simulink model "brake_press_ex"  (R2023b)
settings: Solver=FixedStepAuto  StartTime=0.0  StopTime=10.0  FixedStep=0.01  RelTol=1e-3
settings Model: Creator=FM22  LastModifiedBy=FM22

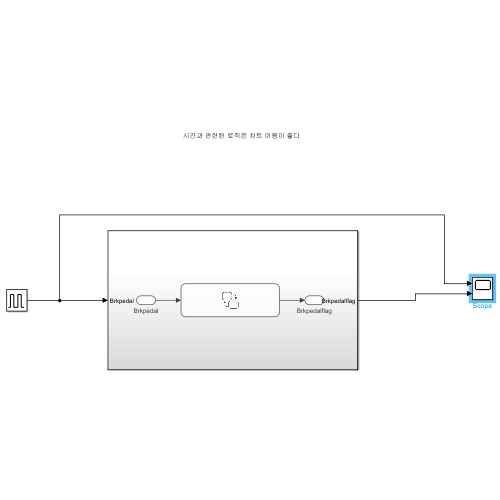
[thumbnail: Simulink's stored preview of the top-level diagram]
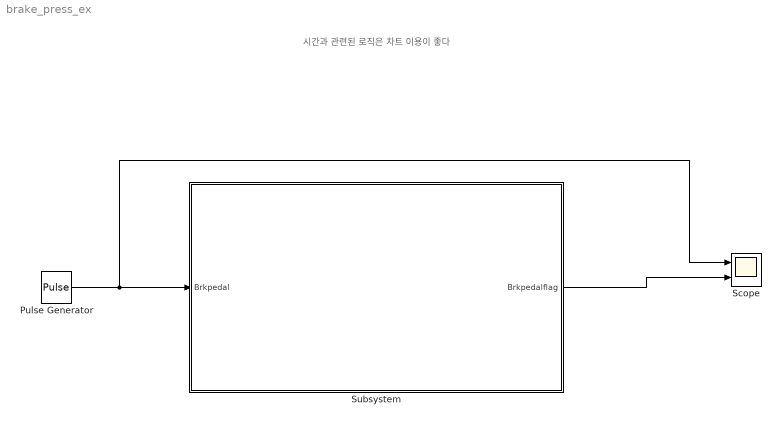
== system brake_press_ex ==
  note: 시간과 관련된 로직은 차트 이용이 좋다
  Pulse Generator : DiscretePulseGenerator  PulseType=Time based  Period=5  PulseWidth=50
  Scope : Scope  NumInputPorts=2
  Subsystem : Subsystem
  wires:
  Pulse Generator/1 -> Scope/1, Subsystem/1(Brkpedal)
  Subsystem/1(Brkpedalflag) -> Scope/2

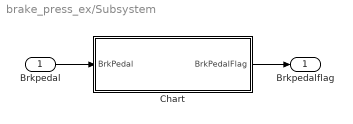
== system brake_press_ex/Subsystem ==
  Brkpedal : Inport
  Chart : Stateflow chart  TreatAsAtomicUnit=on
  Brkpedalflag : Outport
  wires:
  Brkpedal/1 -> Chart/1(BrkPedal)
  Chart/1(BrkPedalFlag) -> Brkpedalflag/1

== stateflow chart brake_press_ex/Subsystem/Chart ==
  state brk_pedal
    en,du:
    press = duration(BrkPedal == 1, msec)>=100;
    unpress = duration(BrkPedal == 0, msec)>=500;
    state UNPRESSED
      BrkPedalFlag = 0;
    state PRESSED
      BrkPedalFlag = 1;
    (default) -> UNPRESSED
    UNPRESSED -> PRESSED : [press]
    PRESSED -> UNPRESSED : [unpress]
  data: BrkPedal input; BrkPedalFlag output; press local; unpress local
